simulink model "Demo2_2"  (R2016a)
settings: Solver=ode45  StartTime=0.0  StopTime=10  MaxStep=0.1  RelTol=1e-3
settings Model: Creator=peter  LastModifiedBy=peter
settings GRTTargetCC: GeneratePreprocessorConditionals=Use local settings

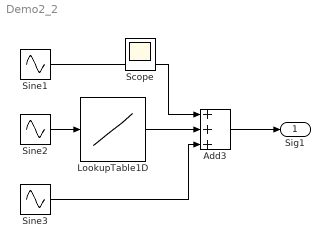
== system Demo2_2 ==
  Add3 : Sum  Inputs=3
  LookupTable1D : Lookup_n-D  NumberOfTableDimensions=1  BreakpointsForDimension1=[-5:5]  Table=tanh([-5:5])  InternalRulePriority=Speed  RndMeth=Simplest  InputSameDT=on
  Sine1 : Sin  Amplitude=0.1  Frequency=1.0472  SampleTime=0
  Sine2 : Sin  Amplitude=2  SampleTime=0
  Sine3 : Sin  Amplitude=0.3  Frequency=0.5236  SampleTime=0
  Sig1 : Outport
  Scope : Scope
  wires:
  Sine1/1 -> Add3/1
  Sine2/1 -> LookupTable1D/1
  Sine3/1 -> Add3/3
  Add3/1 -> Sig1/1
  LookupTable1D/1 -> Add3/2
